simulink model "simulink_lyapunov_R2020a"  (R2020a)
settings: Solver=ode4  StartTime=0.0  StopTime=4  FixedStep=0.01  RelTol=1e-3  EnableMultiTasking=on
values from neighbouring files (symbols this model uses):
  A = [ 0 -5 ... (first row only)    [lyapunov_lyap.m]    (also in lyapunov_lyap2.m)
  P = lyap(A',Q)    [lyapunov_lyap.m]    (also in lyapunov_lyap2.m)
  x0 = [ 1  0 ]'    [run_simulink.m]    (also in run_simulink2.m)
settings Model: Creator=kawata  LastModifiedBy=kawata
settings DataIOCC: LimitDataPoints=on  SaveFormat=Array  SignalLoggingSaveFormat=ModelDataLogs  ReturnWorkspaceOutputs=off
settings OptimizationCC: ExpressionDepthLimit=2147483647  LifeSpan=inf
settings DebuggingCC: UnderspecifiedInitializationDetection=Classic  MergeDetectMultiDrivingBlocksExec=none  SolverPrmCheckMsg=warning  FcnCallInpInsideContextMsg=warning  StateNameClashWarn=warning  SFUnexpectedBacktrackingDiag=warning  SFNoUnconditionalDefaultTransitionDiag=warning  SFExecutionAtInitializationDiag=none  ArithmeticOperatorsInVariantConditions=warning
settings HardwareCC: ProdBitPerPointer=32  ProdBitPerSizeT=32  ProdBitPerPtrDiffT=32  ProdLargestAtomicFloat=None  ProdIntDivRoundTo=Undefined  ProdEndianess=Unspecified  ProdWordSize=32  ProdHWDeviceType=32-bit Generic
settings ModelReferenceCC: PropagateSignalLabelsOutOfModel=off
settings SFSimCC: SimUseLocalCustomCode=off  CustomCodeUndefinedFunction=UseInterfaceOnly
settings RTWCC: RTWUseLocalCustomCode=off
settings CodeAppCC: StateflowObjectComments=on
settings GRTTargetCC: TargetLangStandard=C89/C90 (ANSI)  CombineOutputUpdateFcns=off  GRTInterface=on
settings ConfigComp: CovMetricSettings=dw  CovSaveCumulativeToWorkspaceVar=on  CovSaveSingleToWorkspaceVar=on  CovExternalEMLEnable=off

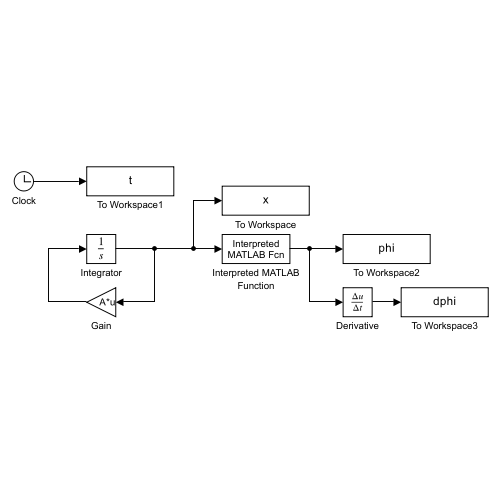
[thumbnail: Simulink's stored preview of the top-level diagram]
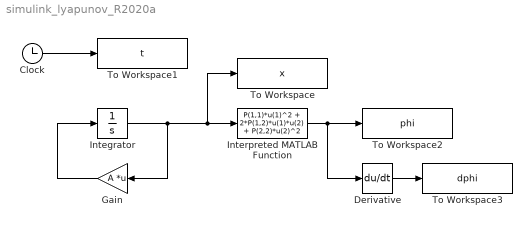
== system simulink_lyapunov_R2020a ==
  Clock : Clock
  Derivative : Derivative
  Gain : Gain  Gain=A  Multiplication=Matrix(K*u)
  Integrator : Integrator  InitialCondition=x0
  Interpreted MATLAB Function : MATLABFcn  MATLABFcn=P(1,1)*u(1)^2 + 2*P(1,2)*u(1)*u(2) + P(2,2)*u(2)^2
  To Workspace : ToWorkspace  VariableName=x  SampleTime=-1
  To Workspace1 : ToWorkspace  VariableName=t  SampleTime=-1
  To Workspace2 : ToWorkspace  VariableName=phi  SampleTime=-1
  To Workspace3 : ToWorkspace  VariableName=dphi  SampleTime=-1
  wires:
  Clock/1 -> To Workspace1/1
  Gain/1 -> Integrator/1
  Integrator/1 -> To Workspace/1, Interpreted MATLAB Function/1, Gain/1
  Interpreted MATLAB Function/1 -> To Workspace2/1, Derivative/1
  Derivative/1 -> To Workspace3/1
